simulink model "mass_spring4"  (R2022b)
settings: Solver=VariableStepAuto  StartTime=0.0  StopTime=Sim_Tim  RelTol=1e-3
undefined symbols (not defined in the file): b1, b2, F, k1, k2, m1, m2
settings Model: Creator=HashimAbdulAzizHashi  LastModifiedBy=HashimAbdulAzizHashi

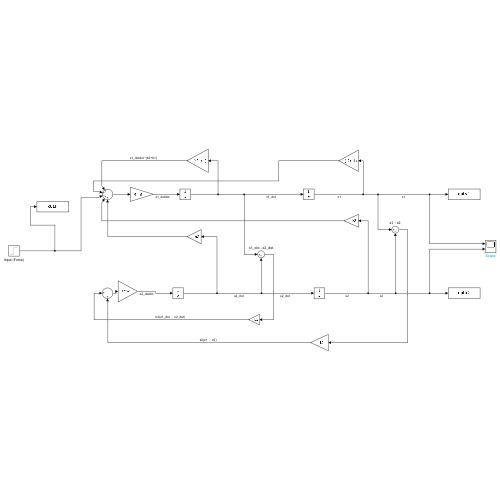
[thumbnail: Simulink's stored preview of the top-level diagram]
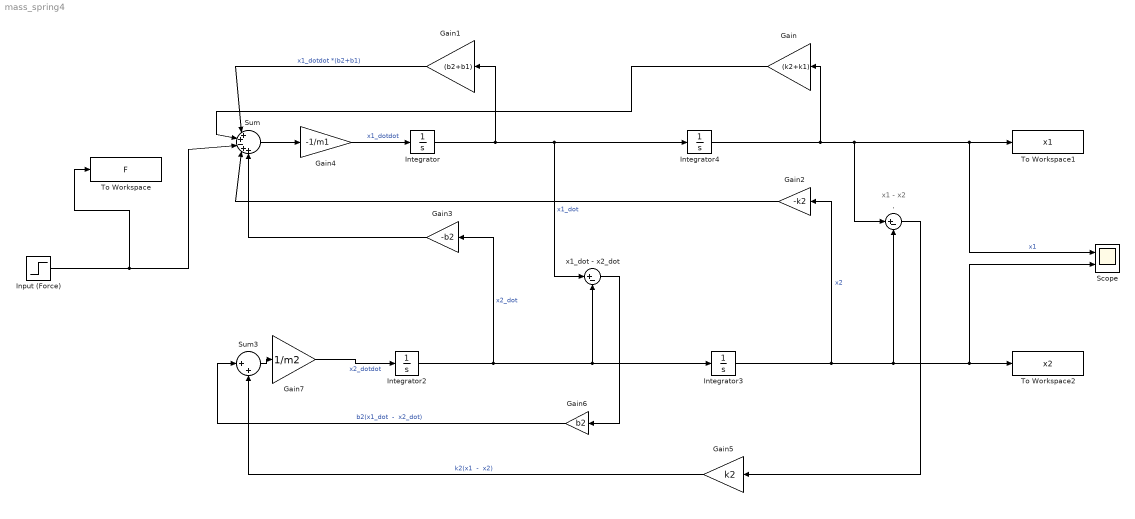
== system mass_spring4 ==
  note: x1 - x2
  . : Sum  Inputs=|+-
  Gain : Gain  Gain=(k2+k1)
  Gain1 : Gain  Gain=(b2+b1)
  Gain2 : Gain  Gain=-k2
  Gain3 : Gain  Gain=-b2
  Gain4 : Gain  Gain=-1/m1
  Gain5 : Gain  Gain=k2
  Gain6 : Gain  Gain=b2
  Gain7 : Gain  Gain=1/m2
  Input (Force) : Step  After=F  SampleTime=0
  Integrator{,2..4} (4 alike) : Integrator
  Scope : Scope  NumInputPorts=2
  Sum : Sum  Inputs=|++-++
  Sum3 : Sum  Inputs=|++
  To Workspace : ToWorkspace  VariableName=F  SaveFormat=Timeseries  SampleTime=-1
  To Workspace1 : ToWorkspace  VariableName=x1  SaveFormat=Timeseries  SampleTime=-1
  To Workspace2 : ToWorkspace  VariableName=x2  SaveFormat=Timeseries  SampleTime=-1
  x1_dot - x2_dot : Sum  Inputs=|+-
  wires:
  Integrator/1 -> Gain1/1, x1_dot - x2_dot/1, Integrator4/1  "x1_dot"
  Integrator2/1 -> Gain3/1, x1_dot - x2_dot/2, Integrator3/1  "x2_dot"
  Gain4/1 -> Integrator/1  "x1_dotdot"
  Integrator4/1 -> Scope/1, To Workspace1/1, ./1, Gain/1  "x1"
  Integrator3/1 -> Gain2/1, Scope/2, To Workspace2/1, ./2  "x2"
  Gain2/1 -> Sum/4
  Gain1/1 -> Sum/1  "x1_dotdot *(b2+b1)"
  Gain/1 -> Sum/2
  Sum/1 -> Gain4/1
  Gain3/1 -> Sum/5
  ./1 -> Gain5/1
  x1_dot - x2_dot/1 -> Gain6/1
  Gain6/1 -> Sum3/1  "b2(x1_dot  -  x2_dot)"
  Gain5/1 -> Sum3/2  "k2(x1  -  x2)"
  Sum3/1 -> Gain7/1
  Gain7/1 -> Integrator2/1  "x2_dotdot"
  Input (Force)/1 -> To Workspace/1, Sum/3
